simulink model "Controller_ABS_VLC_AYC_ALGO2"  (Simulink 8.7)
settings: Solver=ode3  SolverMode=SingleTasking  StartTime=0.0  StopTime=6  FixedStep=0.001  RelTol=1e-3
undefined symbols (not defined in the file): Cf, Cr, g, Lat_Accel_Err_Gain, Lf, Lr, PWM_Low_Lim, PWM_SW_Threshold, Slip_Err_D_Gain, Slip_Err_P_Gain, T_Avail, Target_SR, Yaw_Ctrl_Gain
libraries: dspfdesign x10
settings Model: MinMaxOverflowLogging=ForceOff  Creator=MR Spyder  LastModifiedBy=MR Spyder
settings DataIOCC: SignalLoggingSaveFormat=ModelDataLogs  SaveOutput=off  SaveTime=off
settings OptimizationCC: DefaultParameterBehavior=Inlined  ExpressionDepthLimit=2147483647
settings DebuggingCC: SolverPrmCheckMsg=warning  FcnCallInpInsideContextMsg=EnableAllAsWarning  StateNameClashWarn=warning
settings GRTTargetCC: CombineOutputUpdateFcns=off  GRTInterface=on

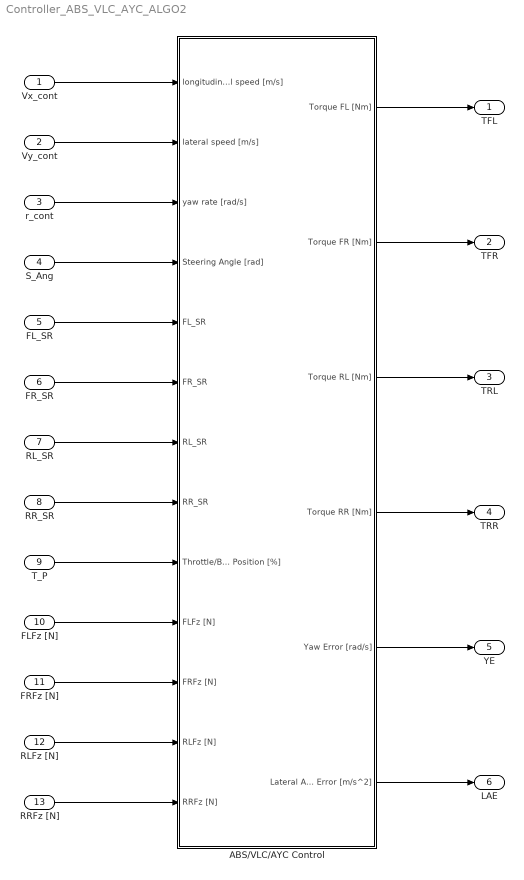
== system Controller_ABS_VLC_AYC_ALGO2 ==
  Vx_cont : Inport
  Vy_cont : Inport  Port=2
  r_cont : Inport  Port=3
  S_Ang : Inport  Port=4
  FL_SR : Inport  Port=5
  FR_SR : Inport  Port=6
  RL_SR : Inport  Port=7
  RR_SR : Inport  Port=8
  T_P : Inport  Port=9
  FLFz [N] : Inport  Port=10
  FRFz [N] : Inport  Port=11
  RLFz [N] : Inport  Port=12
  RRFz [N] : Inport  Port=13
  ABS/VLC/AYC Control : Subsystem
  TFL : Outport
  TFR : Outport  Port=2
  TRL : Outport  Port=3
  TRR : Outport  Port=4
  YE : Outport  Port=5
  LAE : Outport  Port=6
  wires:
  T_P/1 -> ABS/VLC/AYC Control/9(Throttle/Brake Position [%])
  ABS/VLC/AYC Control/1(Torque FL [Nm]) -> TFL/1
  ABS/VLC/AYC Control/2(Torque FR [Nm]) -> TFR/1
  ABS/VLC/AYC Control/3(Torque RL [Nm]) -> TRL/1
  ABS/VLC/AYC Control/4(Torque RR [Nm]) -> TRR/1
  FL_SR/1 -> ABS/VLC/AYC Control/5(FL_SR)
  FR_SR/1 -> ABS/VLC/AYC Control/6(FR_SR)
  RL_SR/1 -> ABS/VLC/AYC Control/7(RL_SR)
  RR_SR/1 -> ABS/VLC/AYC Control/8(RR_SR)
  r_cont/1 -> ABS/VLC/AYC Control/3(yaw rate [rad/s])
  Vy_cont/1 -> ABS/VLC/AYC Control/2(lateral speed [m/s])
  Vx_cont/1 -> ABS/VLC/AYC Control/1(longitudinal speed [m/s])
  S_Ang/1 -> ABS/VLC/AYC Control/4(Steering Angle [rad])
  ABS/VLC/AYC Control/5(Yaw Error [rad/s]) -> YE/1
  FLFz [N]/1 -> ABS/VLC/AYC Control/10(FLFz [N])
  FRFz [N]/1 -> ABS/VLC/AYC Control/11(FRFz [N])
  RLFz [N]/1 -> ABS/VLC/AYC Control/12(RLFz [N])
  RRFz [N]/1 -> ABS/VLC/AYC Control/13(RRFz [N])
  ABS/VLC/AYC Control/6(Lateral Accel Error [m/s^2]) -> LAE/1

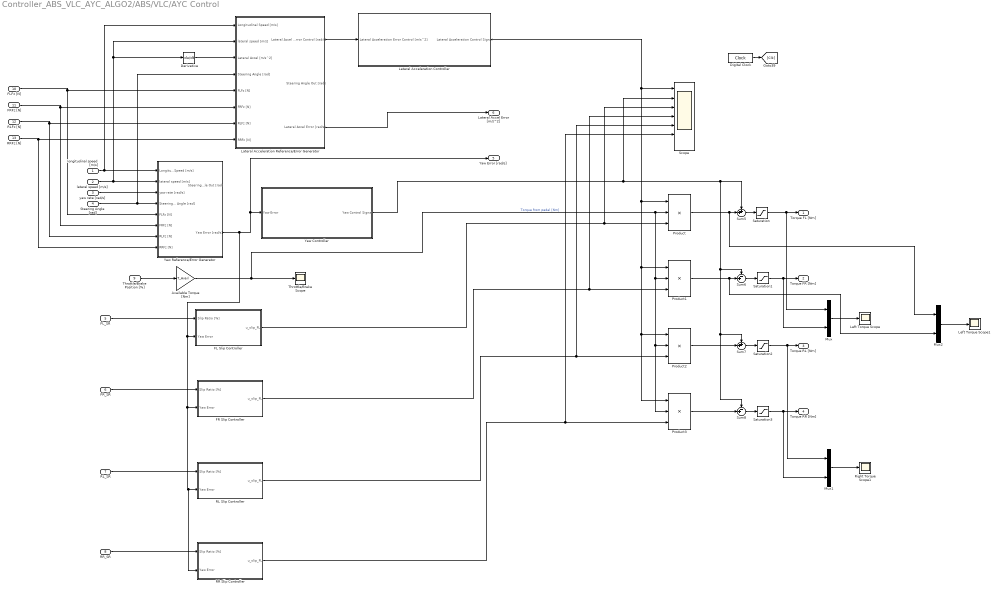
== system Controller_ABS_VLC_AYC_ALGO2/ABS/VLC/AYC Control ==
  longitudinal speed [m/s] : Inport
  lateral speed [m/s] : Inport  Port=2
  yaw rate [rad/s] : Inport  Port=3
  Steering Angle [rad] : Inport  Port=4
  FL_SR : Inport  Port=5
  FR_SR : Inport  Port=6
  RL_SR : Inport  Port=7
  RR_SR : Inport  Port=8
  Throttle/Brake Position [%] : Inport  Port=9
  FLFz [N] : Inport  Port=10
  FRFz [N] : Inport  Port=11
  RLFz [N] : Inport  Port=12
  RRFz [N] : Inport  Port=13
  Available Torque [Nm] : Gain  Gain=T_Avail
  Derivative : Derivative
  Digital Clock : DigitalClock  SampleTime=0.001
  FL Slip Controller : Subsystem
  FR Slip Controller : Subsystem
  Lateral Acceleration Controller : Subsystem
  Lateral Acceleration Reference/Error Generator : Subsystem
  Left Torque Scope : Scope
  Left Torque Scope1 : Scope
  Mux : Mux  Inputs=2
  Mux1 : Mux  Inputs=2
  Mux2 : Mux  Inputs=2
  Product{,1..3} (4 alike) : Product  Inputs=3
  RL Slip Controller : Subsystem
  RR Slip Controller : Subsystem
  Right Torque Scope1 : Scope
  Saturation{,1..3} (4 alike) : Saturate  UpperLimit=150  LowerLimit=-150  LinearizeAsGain=off
  Scope : Scope  NumInputPorts=7
  Sum5 : Sum  Inputs=++|
  Sum6 : Sum  Inputs=-+|
  Sum7 : Sum  Inputs=++|
  Sum8 : Sum  Inputs=-+|
  Throttle/Brake Scope : Scope
  Yaw Controller : Subsystem
  Yaw Reference/Error Generator : Subsystem
  Torque FL [Nm] : Outport
  Torque FR [Nm] : Outport  Port=2
  Torque RL [Nm] : Outport  Port=3
  Torque RR [Nm] : Outport  Port=4
  Yaw Error [rad/s] : Outport  Port=5
  Lateral Accel Error [m/s^2] : Outport  Port=6
  wires:
  Mux/1 -> Left Torque Scope/1
  longitudinal speed [m/s]/1 -> Lateral Acceleration Reference/Error Generator/1(Longitudinal Speed [m/s]), Yaw Reference/Error Generator/1(Longitudinal Speed [m/s])
  lateral speed [m/s]/1 -> Yaw Reference/Error Generator/2(lateral speed [m/s]), Lateral Acceleration Reference/Error Generator/2(lateral speed [m/s]), Derivative/1
  yaw rate [rad/s]/1 -> Yaw Reference/Error Generator/3(yaw rate [rad/s])
  Steering Angle [rad]/1 -> Yaw Reference/Error Generator/4(Steering Angle [rad]), Lateral Acceleration Reference/Error Generator/4(Steering Angle [rad])
  Throttle/Brake Position [%]/1 -> Available Torque [Nm]/1
  Available Torque [Nm]/1 -> Product3/2, Product2/2, Product1/2, Product/2, Throttle/Brake Scope/1  "Torque from pedal [Nm]"
  Mux1/1 -> Right Torque Scope1/1
  FL_SR/1 -> FL Slip Controller/1(Slip Ratio [%])
  FR_SR/1 -> FR Slip Controller/1(Slip Ratio [%])
  RL_SR/1 -> RL Slip Controller/1(Slip Ratio [%])
  RR_SR/1 -> RR Slip Controller/1(Slip Ratio [%])
  Digital Clock/1 -> [Clk]
  FLFz [N]/1 -> Yaw Reference/Error Generator/5(FLFz [N]), Lateral Acceleration Reference/Error Generator/5(FLFz [N])
  FRFz [N]/1 -> Yaw Reference/Error Generator/6(FRFz [N]), Lateral Acceleration Reference/Error Generator/6(FRFz [N])
  RLFz [N]/1 -> Yaw Reference/Error Generator/7(RLFz [N]), Lateral Acceleration Reference/Error Generator/7(RLFz [N])
  RRFz [N]/1 -> Yaw Reference/Error Generator/8(RRFz [N]), Lateral Acceleration Reference/Error Generator/8(RRFz [N])
  Lateral Acceleration Reference/Error Generator/1(Lateral Accel Error Control [rad/s]) -> Lateral Acceleration Controller/1(Lateral Acceleration Error Control [m/s^2])
  Product2/1 -> Sum7/2
  Product3/1 -> Sum8/2
  Sum5/1 -> Saturation/1
  Sum6/1 -> Saturation1/1
  Sum7/1 -> Saturation2/1
  Sum8/1 -> Saturation3/1
  Yaw Reference/Error Generator/2(Yaw Error [rad/s]) -> RR Slip Controller/2(Yaw Error), RL Slip Controller/2(Yaw Error), FR Slip Controller/2(Yaw Error), FL Slip Controller/2(Yaw Error), Yaw Error [rad/s]/1, Yaw Controller/1(Yaw Error)
  Derivative/1 -> Lateral Acceleration Reference/Error Generator/3(Lateral Accel [m/s^2])
  Lateral Acceleration Controller/1(Lateral Acceleration Control Signal) -> Product1/1, Product2/1, Product3/1, Product/1, Scope/1
  Yaw Controller/1(Yaw Control Signal) -> Scope/2, Sum5/1, Sum7/1, Sum8/1, Sum6/1
  Saturation/1 -> Torque FL [Nm]/1, Mux/1
  Saturation1/1 -> Torque FR [Nm]/1, Mux/2
  Saturation2/1 -> Torque RL [Nm]/1, Mux1/1
  Saturation3/1 -> Torque RR [Nm]/1, Mux1/2
  Lateral Acceleration Reference/Error Generator/3(Lateral Accel Error [rad/s]) -> Lateral Accel Error [m/s^2]/1
  Mux2/1 -> Left Torque Scope1/1
  Product/1 -> Mux2/1, Sum5/2
  Product1/1 -> Mux2/2, Sum6/2
  FL Slip Controller/1(u_slip_FL) -> Scope/3, Product/3
  FR Slip Controller/1(u_slip_FL) -> Scope/4, Product1/3
  RL Slip Controller/1(u_slip_FL) -> Scope/5, Product2/3
  RR Slip Controller/1(u_slip_FL) -> Scope/6, Product3/3

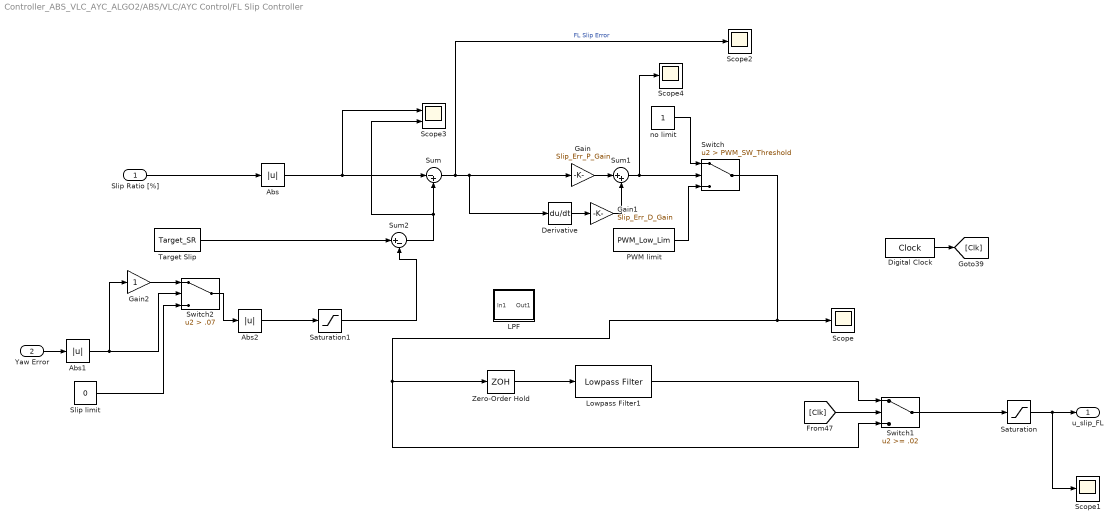
== system Controller_ABS_VLC_AYC_ALGO2/ABS/VLC/AYC Control/FL Slip Controller ==
  Slip Ratio [%] : Inport
  Yaw Error : Inport  Port=2
  Abs : Abs
  Abs1 : Abs
  Abs2 : Abs
  Derivative : Derivative
  Digital Clock : DigitalClock  SampleTime=0.001
  Gain : Gain  Gain=Slip_Err_P_Gain
  Gain1 : Gain  Gain=Slip_Err_D_Gain
  Gain2 : Gain
  LPF : Subsystem
  Lowpass Filter1 : dspfdesign/Lowpass Filter  FilterType=FIR  DesignForMinimumOrder=on  FilterOrder=50  PassbandFrequency=Slip_Pass_Band  StopbandFrequency=Slip_Stop_Band  PassbandRipple=0.1  StopbandAttenuation=80  InheritSampleRate=on  SampleRate=1000  roundingMode=Floor  coeffsDataTypeStr=fixdt(1,16)  SimulateUsing=Interpreted execution
  PWM limit : Constant  Value=PWM_Low_Lim
  Saturation : Saturate  UpperLimit=1  LowerLimit=0
  Saturation1 : Saturate  UpperLimit=Target_SR  LowerLimit=0
  Scope{,1..2,4} (4 alike) : Scope
  Scope3 : Scope  NumInputPorts=2
  Slip limit : Constant  Value=0
  Sum : Sum  Inputs=|-+
  Sum1 : Sum  Inputs=|++
  Sum2 : Sum  Inputs=|+-
  Switch : Switch  Criteria=u2 > Threshold  Threshold=PWM_SW_Threshold
  Switch1 : Switch  Threshold=.02
  Switch2 : Switch  Criteria=u2 > Threshold  Threshold=.07
  Target Slip : Constant  Value=Target_SR
  Zero-Order Hold : ZeroOrderHold  SampleTime=.001
  no limit : Constant
  u_slip_FL : Outport
  wires:
  Target Slip/1 -> Sum2/1
  Sum/1 -> Scope2/1, Derivative/1, Gain/1  "FL Slip Error"
  Derivative/1 -> Gain1/1
  Gain/1 -> Sum1/1
  Sum1/1 -> Scope4/1, Switch/2
  no limit/1 -> Switch/1
  PWM limit/1 -> Switch/3
  Slip Ratio [%]/1 -> Abs/1
  [Clk] -> Switch1/2
  Digital Clock/1 -> [Clk]
  Saturation/1 -> Scope1/1, u_slip_FL/1
  Yaw Error/1 -> Abs1/1
  Sum2/1 -> Scope3/2, Sum/2
  Slip limit/1 -> Switch2/3
  Gain2/1 -> Switch2/1
  Abs1/1 -> Gain2/1, Switch2/2
  Lowpass Filter1/1 -> Switch1/1
  Abs/1 -> Sum/1, Scope3/1
  Switch2/1 -> Abs2/1
  Gain1/1 -> Sum1/2
  Zero-Order Hold/1 -> Lowpass Filter1/1
  Switch/1 -> Zero-Order Hold/1, Switch1/3, Scope/1
  Abs2/1 -> Saturation1/1
  Saturation1/1 -> Sum2/2
  Switch1/1 -> Saturation/1

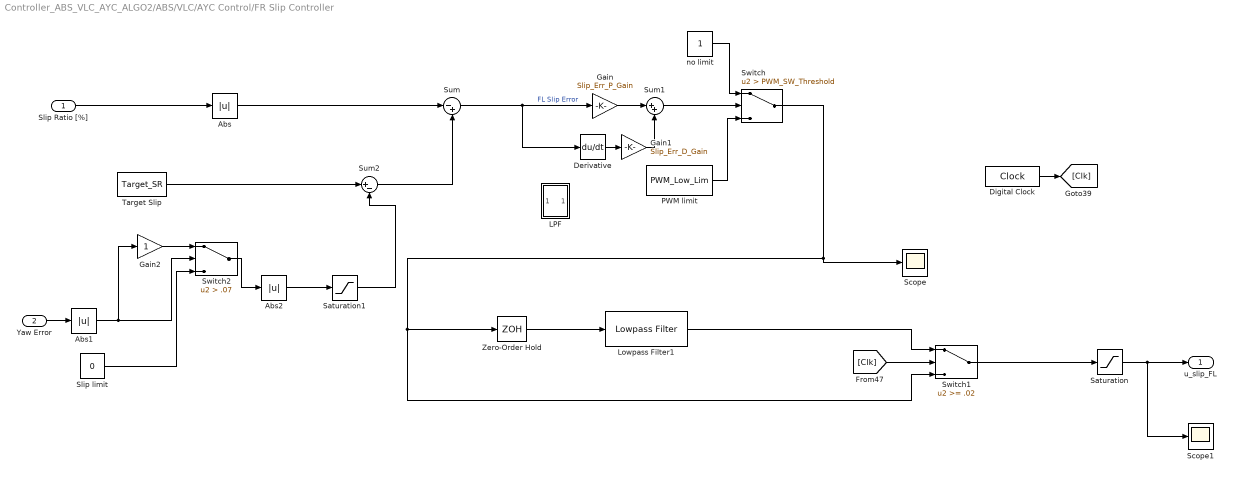
== system Controller_ABS_VLC_AYC_ALGO2/ABS/VLC/AYC Control/FR Slip Controller ==
  Slip Ratio [%] : Inport
  Yaw Error : Inport  Port=2
  Abs : Abs
  Abs1 : Abs
  Abs2 : Abs
  Derivative : Derivative
  Digital Clock : DigitalClock  SampleTime=0.001
  Gain : Gain  Gain=Slip_Err_P_Gain
  Gain1 : Gain  Gain=Slip_Err_D_Gain
  Gain2 : Gain
  LPF : Subsystem
  Lowpass Filter1 : dspfdesign/Lowpass Filter  FilterType=FIR  DesignForMinimumOrder=on  FilterOrder=50  PassbandFrequency=Slip_Pass_Band  StopbandFrequency=Slip_Stop_Band  PassbandRipple=0.1  StopbandAttenuation=80  InheritSampleRate=on  SampleRate=1000  roundingMode=Floor  coeffsDataTypeStr=fixdt(1,16)  SimulateUsing=Interpreted execution
  PWM limit : Constant  Value=PWM_Low_Lim
  Saturation : Saturate  UpperLimit=1  LowerLimit=0
  Saturation1 : Saturate  UpperLimit=Target_SR  LowerLimit=0
  Scope : Scope
  Scope1 : Scope
  Slip limit : Constant  Value=0
  Sum : Sum  Inputs=|-+
  Sum1 : Sum  Inputs=|++
  Sum2 : Sum  Inputs=|+-
  Switch : Switch  Criteria=u2 > Threshold  Threshold=PWM_SW_Threshold
  Switch1 : Switch  Threshold=.02
  Switch2 : Switch  Criteria=u2 > Threshold  Threshold=.07
  Target Slip : Constant  Value=Target_SR
  Zero-Order Hold : ZeroOrderHold  SampleTime=.001
  no limit : Constant
  u_slip_FL : Outport
  wires:
  Sum/1 -> Derivative/1, Gain/1  "FL Slip Error"
  Derivative/1 -> Gain1/1
  Gain/1 -> Sum1/1
  Sum1/1 -> Switch/2
  no limit/1 -> Switch/1
  PWM limit/1 -> Switch/3
  [Clk] -> Switch1/2
  Switch1/1 -> Saturation/1
  Digital Clock/1 -> [Clk]
  Saturation/1 -> Scope1/1, u_slip_FL/1
  Yaw Error/1 -> Abs1/1
  Slip limit/1 -> Switch2/3
  Gain2/1 -> Switch2/1
  Abs1/1 -> Gain2/1, Switch2/2
  Sum2/1 -> Sum/2
  Lowpass Filter1/1 -> Switch1/1
  Slip Ratio [%]/1 -> Abs/1
  Target Slip/1 -> Sum2/1
  Abs/1 -> Sum/1
  Switch2/1 -> Abs2/1
  Gain1/1 -> Sum1/2
  Zero-Order Hold/1 -> Lowpass Filter1/1
  Switch/1 -> Zero-Order Hold/1, Switch1/3, Scope/1
  Abs2/1 -> Saturation1/1
  Saturation1/1 -> Sum2/2

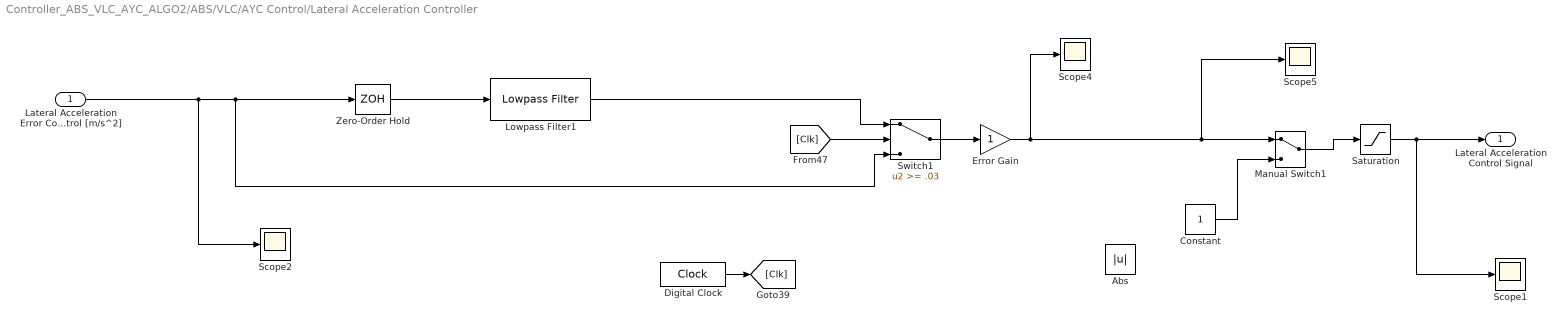
== system Controller_ABS_VLC_AYC_ALGO2/ABS/VLC/AYC Control/Lateral Acceleration Controller ==
  Lateral Acceleration Error Control [m/s^2] : Inport
  Abs : Abs
  Constant : Constant
  Digital Clock : DigitalClock  SampleTime=0.001
  Error Gain : Gain
  Lowpass Filter1 : dspfdesign/Lowpass Filter  FilterType=FIR  DesignForMinimumOrder=on  FilterOrder=50  PassbandFrequency=200  StopbandFrequency=250  PassbandRipple=0.1  StopbandAttenuation=80  InheritSampleRate=on  SampleRate=1000  roundingMode=Floor  coeffsDataTypeStr=fixdt(1,16)  SimulateUsing=Interpreted execution
  Manual Switch1 : ManualSwitch
  Saturation : Saturate  UpperLimit=1  LowerLimit=0
  Scope{1..2,4..5} (4 alike) : Scope
  Switch1 : Switch  Threshold=.03
  Zero-Order Hold : ZeroOrderHold  SampleTime=.001
  Lateral Acceleration Control Signal : Outport
  wires:
  Lateral Acceleration Error Control [m/s^2]/1 -> Scope2/1, Zero-Order Hold/1, Switch1/3
  [Clk] -> Switch1/2
  Lowpass Filter1/1 -> Switch1/1
  Switch1/1 -> Error Gain/1
  Digital Clock/1 -> [Clk]
  Error Gain/1 -> Manual Switch1/1, Scope5/1, Scope4/1
  Saturation/1 -> Scope1/1, Lateral Acceleration Control Signal/1
  Manual Switch1/1 -> Saturation/1
  Constant/1 -> Manual Switch1/2
  Zero-Order Hold/1 -> Lowpass Filter1/1

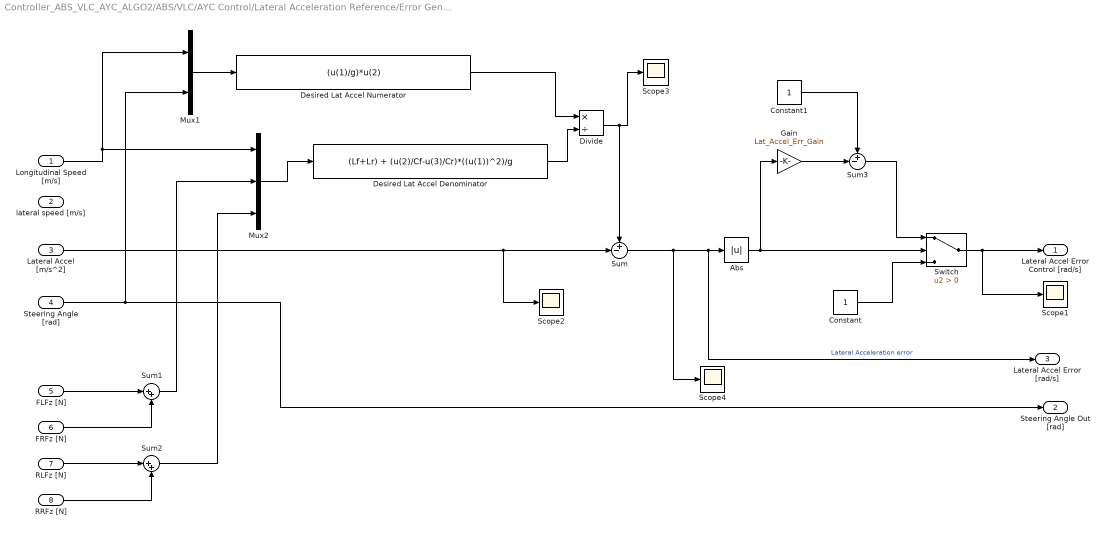
== system Controller_ABS_VLC_AYC_ALGO2/ABS/VLC/AYC Control/Lateral Acceleration Reference/Error Generator ==
  Longitudinal Speed [m/s] : Inport
  lateral speed [m/s] : Inport  Port=2
  Lateral Accel [m/s^2] : Inport  Port=3
  Steering Angle [rad] : Inport  Port=4
  FLFz [N] : Inport  Port=5
  FRFz [N] : Inport  Port=6
  RLFz [N] : Inport  Port=7
  RRFz [N] : Inport  Port=8
  Abs : Abs
  Constant : Constant
  Constant1 : Constant
  Desired Lat Accel Denominator : Fcn  Expr=(Lf+Lr) + (u(2)/Cf-u(3)/Cr)*((u(1))^2)/g
  Desired Lat Accel Numerator : Fcn  Expr=(u(1)/g)*u(2)
  Divide : Product  Inputs=*/
  Gain : Gain  Gain=Lat_Accel_Err_Gain
  Mux1 : Mux  Inputs=2
  Mux2 : Mux  Inputs=3
  Scope{1..4} (4 alike) : Scope
  Sum : Sum  Inputs=+-|
  Sum1 : Sum  Inputs=|++
  Sum2 : Sum  Inputs=|++
  Sum3 : Sum  Inputs=+-|
  Switch : Switch  Criteria=u2 > Threshold
  Lateral Accel Error Control [rad/s] : Outport
  Steering Angle Out [rad] : Outport  Port=2
  Lateral Accel Error [rad/s] : Outport  Port=3
  wires:
  Mux2/1 -> Desired Lat Accel Denominator/1
  Longitudinal Speed [m/s]/1 -> Mux1/1, Mux2/1
  Steering Angle [rad]/1 -> Mux1/2, Steering Angle Out [rad]/1
  Lateral Accel [m/s^2]/1 -> Scope2/1, Sum/2
  Sum/1 -> Scope4/1, Lateral Accel Error [rad/s]/1, Abs/1  "Lateral Acceleration error"
  Desired Lat Accel Numerator/1 -> Divide/1
  Mux1/1 -> Desired Lat Accel Numerator/1
  FLFz [N]/1 -> Sum1/1
  FRFz [N]/1 -> Sum1/2
  Sum1/1 -> Mux2/2
  RLFz [N]/1 -> Sum2/1
  RRFz [N]/1 -> Sum2/2
  Sum2/1 -> Mux2/3
  Desired Lat Accel Denominator/1 -> Divide/2
  Divide/1 -> Scope3/1, Sum/1
  Switch/1 -> Lateral Accel Error Control [rad/s]/1, Scope1/1
  Constant/1 -> Switch/3
  Abs/1 -> Gain/1, Switch/2
  Constant1/1 -> Sum3/1
  Sum3/1 -> Switch/1
  Gain/1 -> Sum3/2

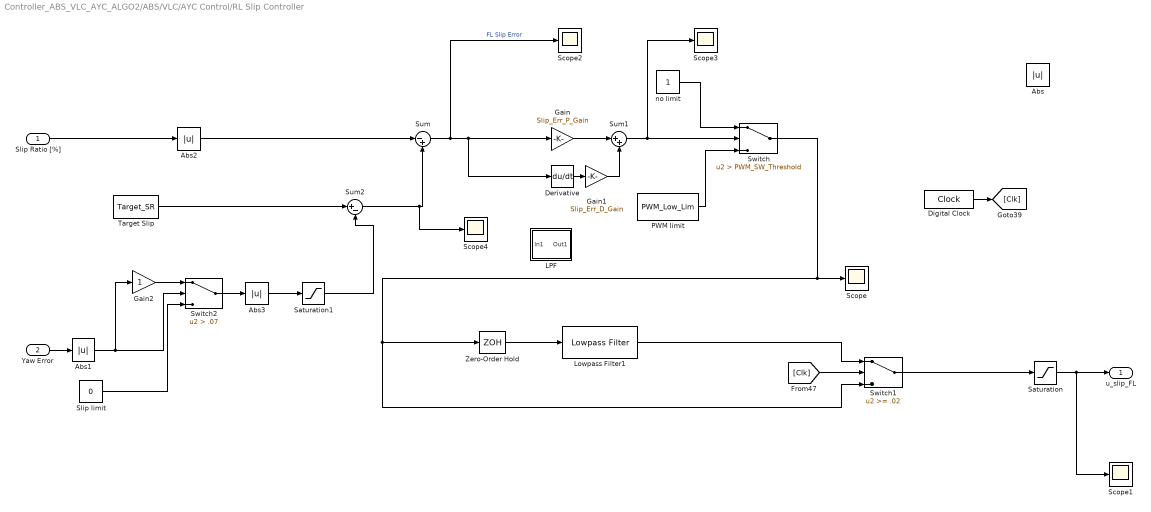
== system Controller_ABS_VLC_AYC_ALGO2/ABS/VLC/AYC Control/RL Slip Controller ==
  Slip Ratio [%] : Inport
  Yaw Error : Inport  Port=2
  Abs{,1..3} (4 alike) : Abs
  Derivative : Derivative
  Digital Clock : DigitalClock  SampleTime=0.001
  Gain : Gain  Gain=Slip_Err_P_Gain
  Gain1 : Gain  Gain=Slip_Err_D_Gain
  Gain2 : Gain
  LPF : Subsystem
  Lowpass Filter1 : dspfdesign/Lowpass Filter  FilterType=FIR  DesignForMinimumOrder=on  FilterOrder=50  PassbandFrequency=Slip_Pass_Band  StopbandFrequency=Slip_Stop_Band  PassbandRipple=0.1  StopbandAttenuation=80  InheritSampleRate=on  SampleRate=1000  roundingMode=Floor  coeffsDataTypeStr=fixdt(1,16)  SimulateUsing=Interpreted execution
  PWM limit : Constant  Value=PWM_Low_Lim
  Saturation : Saturate  UpperLimit=1  LowerLimit=0
  Saturation1 : Saturate  UpperLimit=Target_SR  LowerLimit=0
  Scope{,1..4} (5 alike) : Scope
  Slip limit : Constant  Value=0
  Sum : Sum  Inputs=|-+
  Sum1 : Sum  Inputs=|++
  Sum2 : Sum  Inputs=|+-
  Switch : Switch  Criteria=u2 > Threshold  Threshold=PWM_SW_Threshold
  Switch1 : Switch  Threshold=.02
  Switch2 : Switch  Criteria=u2 > Threshold  Threshold=.07
  Target Slip : Constant  Value=Target_SR
  Zero-Order Hold : ZeroOrderHold  SampleTime=.001
  no limit : Constant
  u_slip_FL : Outport
  wires:
  Sum/1 -> Scope2/1, Derivative/1, Gain/1  "FL Slip Error"
  Derivative/1 -> Gain1/1
  Gain/1 -> Sum1/1
  Sum1/1 -> Scope3/1, Switch/2
  no limit/1 -> Switch/1
  PWM limit/1 -> Switch/3
  [Clk] -> Switch1/2
  Switch1/1 -> Saturation/1
  Digital Clock/1 -> [Clk]
  Saturation/1 -> Scope1/1, u_slip_FL/1
  Yaw Error/1 -> Abs1/1
  Slip limit/1 -> Switch2/3
  Gain2/1 -> Switch2/1
  Abs1/1 -> Gain2/1, Switch2/2
  Sum2/1 -> Scope4/1, Sum/2
  Lowpass Filter1/1 -> Switch1/1
  Slip Ratio [%]/1 -> Abs2/1
  Target Slip/1 -> Sum2/1
  Abs2/1 -> Sum/1
  Switch2/1 -> Abs3/1
  Gain1/1 -> Sum1/2
  Zero-Order Hold/1 -> Lowpass Filter1/1
  Switch/1 -> Zero-Order Hold/1, Switch1/3, Scope/1
  Abs3/1 -> Saturation1/1
  Saturation1/1 -> Sum2/2

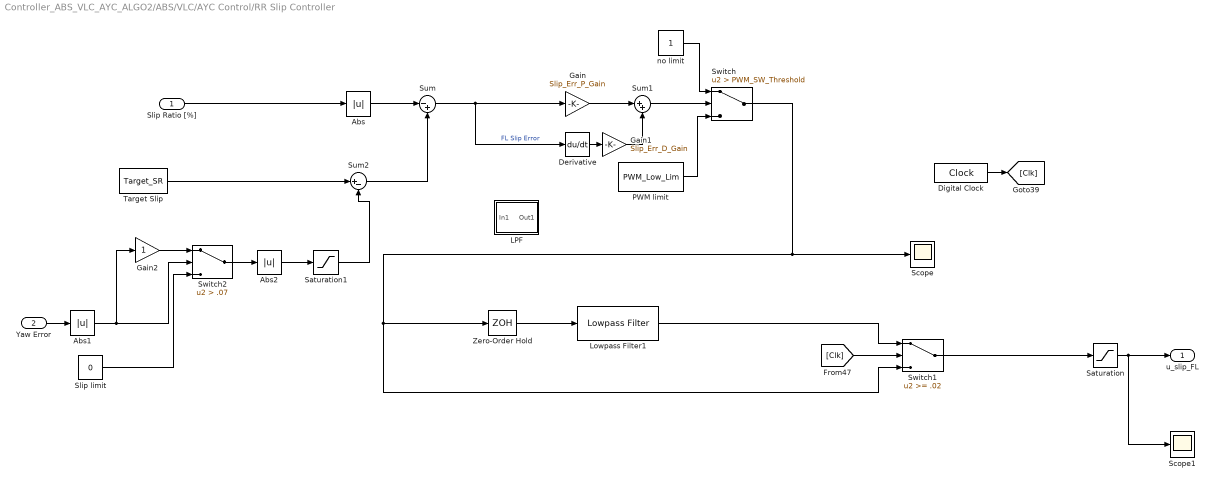
== system Controller_ABS_VLC_AYC_ALGO2/ABS/VLC/AYC Control/RR Slip Controller ==
  Slip Ratio [%] : Inport
  Yaw Error : Inport  Port=2
  Abs : Abs
  Abs1 : Abs
  Abs2 : Abs
  Derivative : Derivative
  Digital Clock : DigitalClock  SampleTime=0.001
  Gain : Gain  Gain=Slip_Err_P_Gain
  Gain1 : Gain  Gain=Slip_Err_D_Gain
  Gain2 : Gain
  LPF : Subsystem
  Lowpass Filter1 : dspfdesign/Lowpass Filter  FilterType=FIR  DesignForMinimumOrder=on  FilterOrder=50  PassbandFrequency=Slip_Pass_Band  StopbandFrequency=Slip_Stop_Band  PassbandRipple=0.1  StopbandAttenuation=80  InheritSampleRate=on  SampleRate=1000  roundingMode=Floor  coeffsDataTypeStr=fixdt(1,16)  SimulateUsing=Interpreted execution
  PWM limit : Constant  Value=PWM_Low_Lim
  Saturation : Saturate  UpperLimit=1  LowerLimit=0
  Saturation1 : Saturate  UpperLimit=Target_SR  LowerLimit=0
  Scope : Scope
  Scope1 : Scope
  Slip limit : Constant  Value=0
  Sum : Sum  Inputs=|-+
  Sum1 : Sum  Inputs=|++
  Sum2 : Sum  Inputs=|+-
  Switch : Switch  Criteria=u2 > Threshold  Threshold=PWM_SW_Threshold
  Switch1 : Switch  Threshold=.02
  Switch2 : Switch  Criteria=u2 > Threshold  Threshold=.07
  Target Slip : Constant  Value=Target_SR
  Zero-Order Hold : ZeroOrderHold  SampleTime=.001
  no limit : Constant
  u_slip_FL : Outport
  wires:
  Sum/1 -> Derivative/1, Gain/1  "FL Slip Error"
  Derivative/1 -> Gain1/1
  Gain/1 -> Sum1/1
  Sum1/1 -> Switch/2
  no limit/1 -> Switch/1
  PWM limit/1 -> Switch/3
  [Clk] -> Switch1/2
  Switch1/1 -> Saturation/1
  Digital Clock/1 -> [Clk]
  Saturation/1 -> Scope1/1, u_slip_FL/1
  Yaw Error/1 -> Abs1/1
  Slip limit/1 -> Switch2/3
  Gain2/1 -> Switch2/1
  Abs1/1 -> Gain2/1, Switch2/2
  Sum2/1 -> Sum/2
  Lowpass Filter1/1 -> Switch1/1
  Slip Ratio [%]/1 -> Abs/1
  Target Slip/1 -> Sum2/1
  Abs/1 -> Sum/1
  Switch2/1 -> Abs2/1
  Gain1/1 -> Sum1/2
  Zero-Order Hold/1 -> Lowpass Filter1/1
  Switch/1 -> Zero-Order Hold/1, Switch1/3, Scope/1
  Abs2/1 -> Saturation1/1
  Saturation1/1 -> Sum2/2

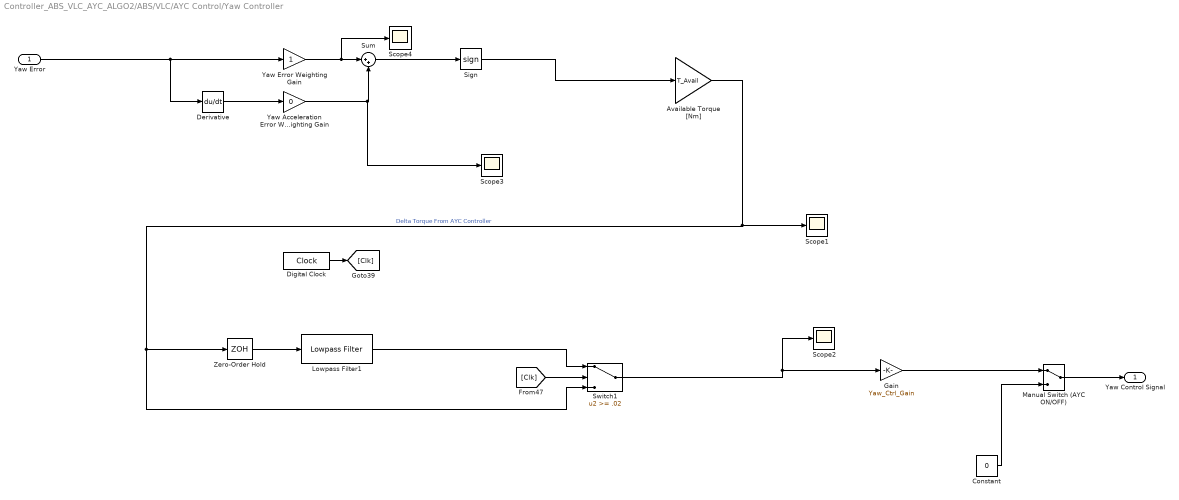
== system Controller_ABS_VLC_AYC_ALGO2/ABS/VLC/AYC Control/Yaw Controller ==
  Yaw Error : Inport
  Available Torque [Nm] : Gain  Gain=T_Avail
  Constant : Constant  Value=0
  Derivative : Derivative
  Digital Clock : DigitalClock  SampleTime=0.001
  Gain : Gain  Gain=Yaw_Ctrl_Gain
  Lowpass Filter1 : dspfdesign/Lowpass Filter  FilterType=FIR  DesignForMinimumOrder=on  FilterOrder=50  PassbandFrequency=200  StopbandFrequency=250  PassbandRipple=0.1  StopbandAttenuation=80  InheritSampleRate=on  SampleRate=1000  roundingMode=Floor  coeffsDataTypeStr=fixdt(1,16)  SimulateUsing=Interpreted execution
  Manual Switch (AYC ON/OFF) : ManualSwitch
  Scope{1..4} (4 alike) : Scope
  Sign : Signum
  Sum : Sum  Inputs=|++
  Switch1 : Switch  Threshold=.02
  Yaw Acceleration Error Weighting Gain : Gain  Gain=0
  Yaw Error Weighting Gain : Gain
  Zero-Order Hold : ZeroOrderHold  SampleTime=.001
  Yaw Control Signal : Outport
  wires:
  Yaw Error Weighting Gain/1 -> Scope4/1, Sum/1
  Yaw Acceleration Error Weighting Gain/1 -> Scope3/1, Sum/2
  Sign/1 -> Available Torque [Nm]/1
  Available Torque [Nm]/1 -> Zero-Order Hold/1, Switch1/3, Scope1/1  "Delta Torque From AYC Controller"
  Derivative/1 -> Yaw Acceleration Error Weighting Gain/1
  [Clk] -> Switch1/2
  Lowpass Filter1/1 -> Switch1/1
  Digital Clock/1 -> [Clk]
  Sum/1 -> Sign/1
  Constant/1 -> Manual Switch (AYC ON/OFF)/2
  Manual Switch (AYC ON/OFF)/1 -> Yaw Control Signal/1
  Yaw Error/1 -> Yaw Error Weighting Gain/1, Derivative/1
  Switch1/1 -> Gain/1, Scope2/1
  Gain/1 -> Manual Switch (AYC ON/OFF)/1
  Zero-Order Hold/1 -> Lowpass Filter1/1

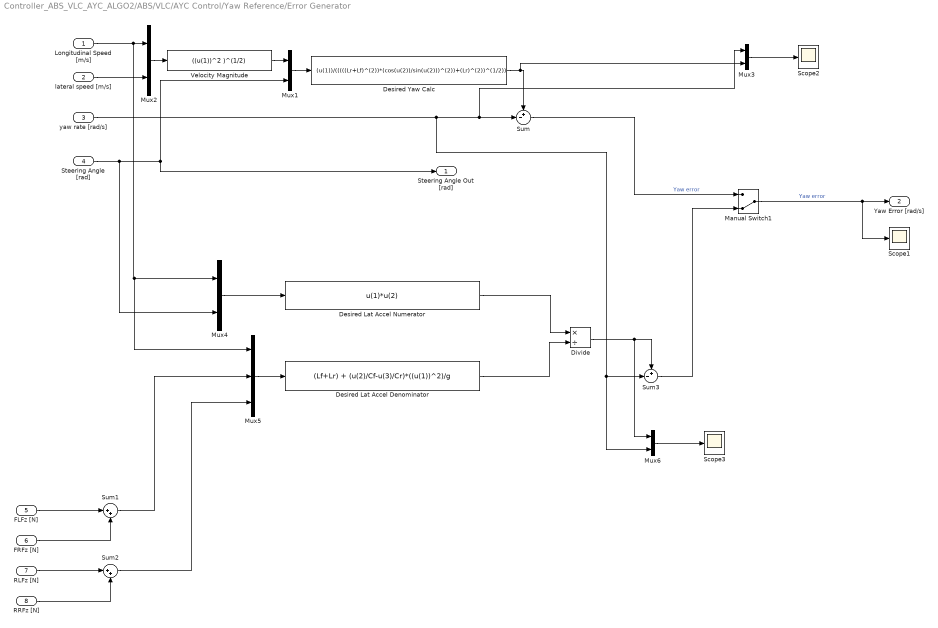
== system Controller_ABS_VLC_AYC_ALGO2/ABS/VLC/AYC Control/Yaw Reference/Error Generator ==
  Longitudinal Speed [m/s] : Inport
  lateral speed [m/s] : Inport  Port=2
  yaw rate [rad/s] : Inport  Port=3
  Steering Angle [rad] : Inport  Port=4
  FLFz [N] : Inport  Port=5
  FRFz [N] : Inport  Port=6
  RLFz [N] : Inport  Port=7
  RRFz [N] : Inport  Port=8
  Desired Lat Accel Denominator : Fcn  Expr=(Lf+Lr) + (u(2)/Cf-u(3)/Cr)*((u(1))^2)/g
  Desired Lat Accel Numerator : Fcn  Expr=u(1)*u(2)
  Desired Yaw Calc : Fcn  Expr=(u(1))/(((((Lr+Lf)^(2))*(cos(u(2))/sin(u(2)))^(2))+(Lr)^(2))^(1/2))
  Divide : Product  Inputs=*/
  Manual Switch1 : ManualSwitch  CurrentSetting=0
  Mux{1..4,6} (5 alike) : Mux  Inputs=2
  Mux5 : Mux  Inputs=3
  Scope1 : Scope
  Scope2 : Scope
  Scope3 : Scope
  Sum : Sum  Inputs=+-|
  Sum1 : Sum  Inputs=|++
  Sum2 : Sum  Inputs=|++
  Sum3 : Sum  Inputs=+-|
  Velocity Magnitude : Fcn  Expr=((u(1))^2 )^(1/2)
  Steering Angle Out [rad] : Outport
  Yaw Error [rad/s] : Outport  Port=2
  wires:
  Mux1/1 -> Desired Yaw Calc/1
  lateral speed [m/s]/1 -> Mux2/2
  Mux2/1 -> Velocity Magnitude/1
  Velocity Magnitude/1 -> Mux1/1
  Steering Angle [rad]/1 -> Mux4/2, Mux1/2, Steering Angle Out [rad]/1
  Desired Yaw Calc/1 -> Sum/1, Mux3/2
  Mux3/1 -> Scope2/1
  Desired Lat Accel Numerator/1 -> Divide/1
  Desired Lat Accel Denominator/1 -> Divide/2
  Longitudinal Speed [m/s]/1 -> Mux5/1, Mux4/1, Mux2/1
  Mux4/1 -> Desired Lat Accel Numerator/1
  FLFz [N]/1 -> Sum1/1
  FRFz [N]/1 -> Sum1/2
  Sum1/1 -> Mux5/2
  RLFz [N]/1 -> Sum2/1
  RRFz [N]/1 -> Sum2/2
  Sum2/1 -> Mux5/3
  Mux5/1 -> Desired Lat Accel Denominator/1
  Manual Switch1/1 -> Yaw Error [rad/s]/1, Scope1/1  "Yaw error"
  Sum/1 -> Manual Switch1/1  "Yaw error"
  Divide/1 -> Mux6/1, Sum3/1
  Sum3/1 -> Manual Switch1/2
  Mux6/1 -> Scope3/1
  yaw rate [rad/s]/1 -> Mux6/2, Sum3/2, Sum/2, Mux3/1

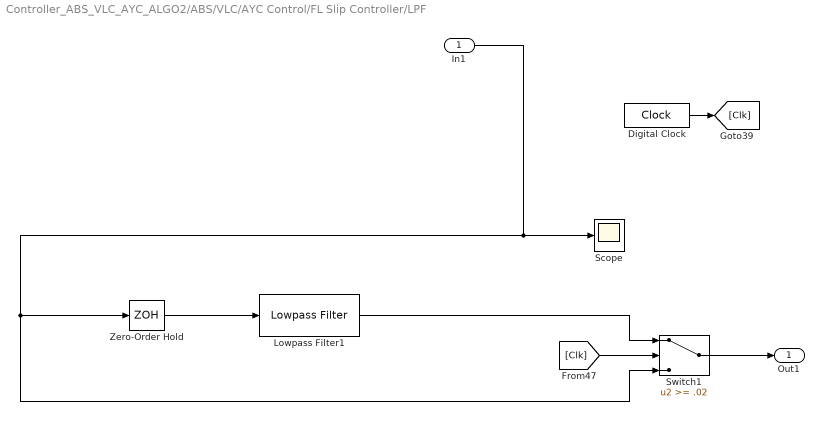
== system Controller_ABS_VLC_AYC_ALGO2/ABS/VLC/AYC Control/FL Slip Controller/LPF ==
  In1 : Inport
  Digital Clock : DigitalClock  SampleTime=0.001
  Lowpass Filter1 : dspfdesign/Lowpass Filter  FilterType=FIR  DesignForMinimumOrder=on  FilterOrder=50  PassbandFrequency=100  StopbandFrequency=150  PassbandRipple=0.1  StopbandAttenuation=80  InheritSampleRate=on  SampleRate=1000  roundingMode=Floor  coeffsDataTypeStr=fixdt(1,16)  SimulateUsing=Interpreted execution
  Scope : Scope
  Switch1 : Switch  Threshold=.02
  Zero-Order Hold : ZeroOrderHold  SampleTime=.001
  Out1 : Outport
  wires:
  In1/1 -> Zero-Order Hold/1, Switch1/3, Scope/1
  [Clk] -> Switch1/2
  Switch1/1 -> Out1/1
  Lowpass Filter1/1 -> Switch1/1
  Digital Clock/1 -> [Clk]
  Zero-Order Hold/1 -> Lowpass Filter1/1

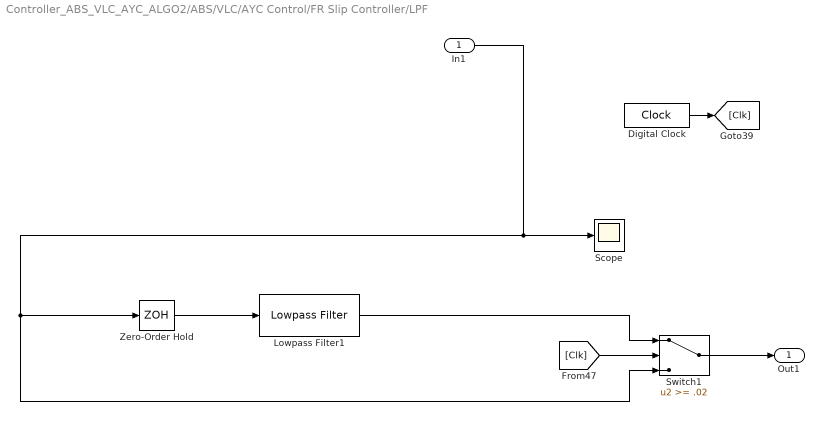
== system Controller_ABS_VLC_AYC_ALGO2/ABS/VLC/AYC Control/FR Slip Controller/LPF ==
  In1 : Inport
  Digital Clock : DigitalClock  SampleTime=0.001
  Lowpass Filter1 : dspfdesign/Lowpass Filter  FilterType=FIR  DesignForMinimumOrder=on  FilterOrder=50  PassbandFrequency=100  StopbandFrequency=150  PassbandRipple=0.1  StopbandAttenuation=80  InheritSampleRate=on  SampleRate=1000  roundingMode=Floor  coeffsDataTypeStr=fixdt(1,16)  SimulateUsing=Interpreted execution
  Scope : Scope
  Switch1 : Switch  Threshold=.02
  Zero-Order Hold : ZeroOrderHold  SampleTime=.001
  Out1 : Outport
  wires:
  In1/1 -> Zero-Order Hold/1, Switch1/3, Scope/1
  [Clk] -> Switch1/2
  Switch1/1 -> Out1/1
  Lowpass Filter1/1 -> Switch1/1
  Digital Clock/1 -> [Clk]
  Zero-Order Hold/1 -> Lowpass Filter1/1

== system Controller_ABS_VLC_AYC_ALGO2/ABS/VLC/AYC Control/RL Slip Controller/LPF ==
  In1 : Inport
  Digital Clock : DigitalClock  SampleTime=0.001
  Lowpass Filter1 : dspfdesign/Lowpass Filter  FilterType=FIR  DesignForMinimumOrder=on  FilterOrder=50  PassbandFrequency=100  StopbandFrequency=150  PassbandRipple=0.1  StopbandAttenuation=80  InheritSampleRate=on  SampleRate=1000  roundingMode=Floor  coeffsDataTypeStr=fixdt(1,16)  SimulateUsing=Interpreted execution
  Scope : Scope
  Switch1 : Switch  Threshold=.02
  Zero-Order Hold : ZeroOrderHold  SampleTime=.001
  Out1 : Outport
  wires:
  In1/1 -> Zero-Order Hold/1, Switch1/3, Scope/1
  [Clk] -> Switch1/2
  Switch1/1 -> Out1/1
  Lowpass Filter1/1 -> Switch1/1
  Digital Clock/1 -> [Clk]
  Zero-Order Hold/1 -> Lowpass Filter1/1

== system Controller_ABS_VLC_AYC_ALGO2/ABS/VLC/AYC Control/RR Slip Controller/LPF ==
  In1 : Inport
  Digital Clock : DigitalClock  SampleTime=0.001
  Lowpass Filter1 : dspfdesign/Lowpass Filter  FilterType=FIR  DesignForMinimumOrder=on  FilterOrder=50  PassbandFrequency=100  StopbandFrequency=150  PassbandRipple=0.1  StopbandAttenuation=80  InheritSampleRate=on  SampleRate=1000  roundingMode=Floor  coeffsDataTypeStr=fixdt(1,16)  SimulateUsing=Interpreted execution
  Scope : Scope
  Switch1 : Switch  Threshold=.02
  Zero-Order Hold : ZeroOrderHold  SampleTime=.001
  Out1 : Outport
  wires:
  In1/1 -> Zero-Order Hold/1, Switch1/3, Scope/1
  [Clk] -> Switch1/2
  Switch1/1 -> Out1/1
  Lowpass Filter1/1 -> Switch1/1
  Digital Clock/1 -> [Clk]
  Zero-Order Hold/1 -> Lowpass Filter1/1
